simulink model "nnsmc_position_HIL"  (R2024b)
settings: Solver=VariableStepAuto  StartTime=0.0  StopTime=0.005  RelTol=1e-3
undefined symbols (not defined in the file or in its folder): CR, LF
libraries: instrumentseriallib x3, stmutilitieslib x1
settings Model: Creator=mohsen  LastModifiedBy=mohsen

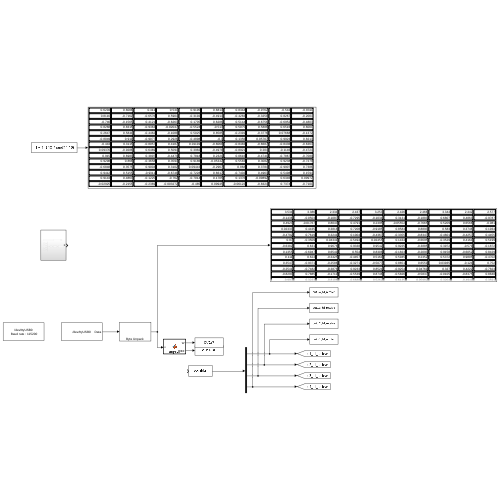
[thumbnail: Simulink's stored preview of the top-level diagram]
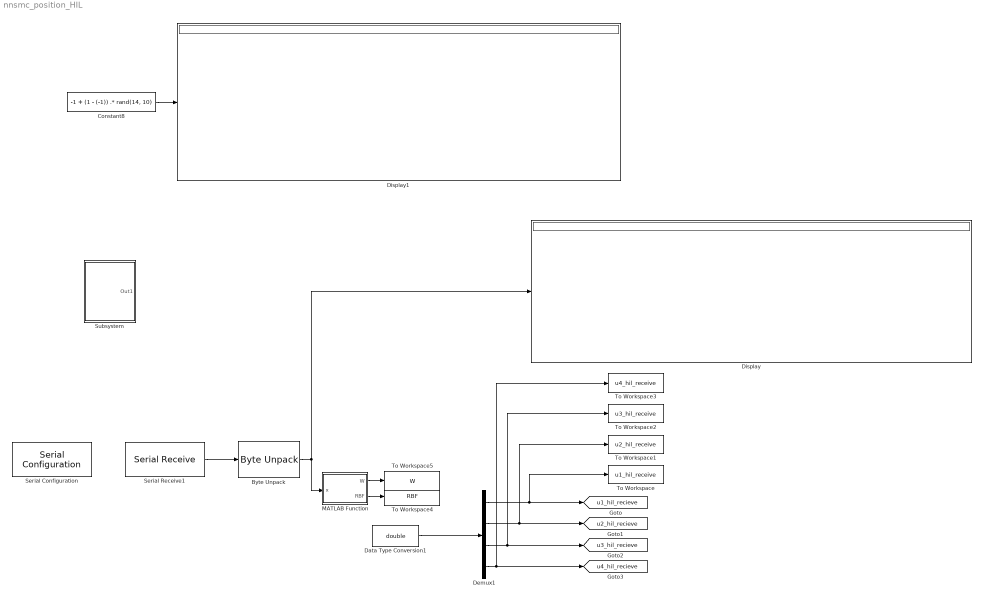
== system nnsmc_position_HIL ==
  Byte Unpack : stmutilitieslib/Byte Unpack  dimensions={[150]}  datatypes={'single'}  byteAlign=1  blockPlatform=stm32f4discovery
  Constant8 : Constant  Value=-1 + (1 - (-1)) .* rand(14, 10)
  Data Type Conversion1 : DataTypeConversion  OutDataTypeStr=double  SaturateOnIntegerOverflow=off  RndMeth=Floor
  Demux1 : Demux
  Display : Display
  Display1 : Display
  MATLAB Function : MATLAB Function  TreatAsAtomicUnit=on
  Serial Configuration : instrumentseriallib/Serial Configuration  Priority=-200000  PortSel=/dev/ttyUSB0  Port=/dev/ttyUSB0  ComPort=/dev/ttyUSB0  BaudRate=115200  DataBits=8  Parity=none  StopBits=1  ByteOrder=little-endian  FlowControl=none  Timeout=0.1  SimulateUsing=Interpreted execution  BlockInModel=on  aMode=1
      settings: LibrarySourceBlock=c2000lib/Host Communication/Serial Configuration
  Serial Receive1 : instrumentseriallib/Serial Receive  Priority=1  PortSel=/dev/ttyUSB0  Port=/dev/ttyUSB0  ComPort=/dev/ttyUSB0  DataType=uint8  SaveDataType=uint8  ToggleHeader=on  Header=[170 187 204]  ToggleDataSize=on  DataSize=600  ToggleTerminator=off  Terminator=CR/LF ('\r\n')  CustomTerminator=[]  InputFormat=Column major  EnableBlockingMode=on  ActionDataUnavailable=Output last received value  ActionWhenDataUnavailable=Output last received value  CustomValue=0  SampleTime=0.005  SimulateUsing=Interpreted execution  BlockInModel=on  aMode=1
      settings: LibrarySourceBlock=c2000lib/Host Communication/Serial Receive
  Subsystem : Subsystem
  To Workspace : ToWorkspace  VariableName=u1_hil_receive  SampleTime=-1
      settings: Save2DSignal=2-D array (concatenate along first dimension)
  To Workspace1 : ToWorkspace  VariableName=u2_hil_receive  SampleTime=-1
      settings: Save2DSignal=2-D array (concatenate along first dimension)
  To Workspace2 : ToWorkspace  VariableName=u3_hil_receive  SampleTime=-1
      settings: Save2DSignal=2-D array (concatenate along first dimension)
  To Workspace3 : ToWorkspace  VariableName=u4_hil_receive  SampleTime=-1
      settings: Save2DSignal=2-D array (concatenate along first dimension)
  To Workspace4 : ToWorkspace  VariableName=RBF  SampleTime=-1
      settings: Save2DSignal=2-D array (concatenate along first dimension)
  To Workspace5 : ToWorkspace  VariableName=W  SampleTime=-1
      settings: Save2DSignal=2-D array (concatenate along first dimension)
  tag scope: u1_hil_recieve=global, u2_hil_recieve=global, u3_hil_recieve=global, u4_hil_recieve=global
  wires:
  Demux1/2 -> To Workspace1/1, [u2_hil_recieve]
  Data Type Conversion1/1 -> Demux1/1
  Demux1/3 -> To Workspace2/1, [u3_hil_recieve]
  Demux1/4 -> To Workspace3/1, [u4_hil_recieve]
  Demux1/1 -> [u1_hil_recieve], To Workspace/1
  Constant8/1 -> Display1/1
  Byte Unpack/1 -> Display/1, MATLAB Function/1(x)
  Serial Receive1/1 -> Byte Unpack/1
  MATLAB Function/2(RBF) -> To Workspace4/1
  MATLAB Function/1(W) -> To Workspace5/1

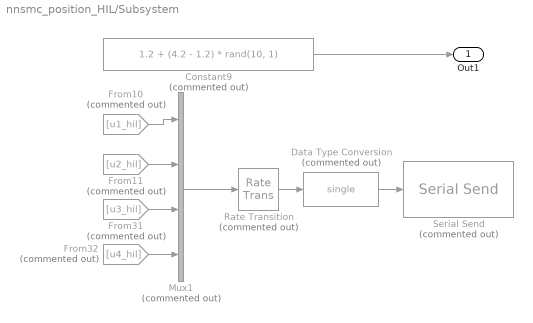
== system nnsmc_position_HIL/Subsystem ==
  Constant9 : Constant  Commented=on  Value=1.2 + (4.2 - 1.2) * rand(10, 1)
  Data Type Conversion : DataTypeConversion  Commented=on  OutDataTypeStr=single  SaturateOnIntegerOverflow=off  RndMeth=Floor
  From10 : From  Commented=on  GotoTag=u1_hil  TagVisibility=global
  From11 : From  Commented=on  GotoTag=u2_hil  TagVisibility=global
  From31 : From  Commented=on  GotoTag=u3_hil  TagVisibility=global
  From32 : From  Commented=on  GotoTag=u4_hil  TagVisibility=global
  Mux1 : Mux  Commented=on
  Rate Transition : RateTransition  Commented=on  OutPortSampleTime=0.005
  Serial Send : instrumentseriallib/Serial Send  Priority=1  Commented=on  PortSel=/dev/ttyUSB0  Port=/dev/ttyUSB0  ComPort=/dev/ttyUSB0  Header=[]  Terminator=<none>  CustomTerminator=[]  EnableBlockingMode=on  SimulateUsing=Interpreted execution  BlockInModel=on  aMode=1
      settings: LibrarySourceBlock=embeddedtargetslib/Host Communication/Serial Send
  Out1 : Outport
  wires:
  Rate Transition/1 -> Data Type Conversion/1
  From31/1 -> Mux1/3
  From10/1 -> Mux1/1
  Constant9/1 -> Out1/1
  From32/1 -> Mux1/4
  From11/1 -> Mux1/2
  Data Type Conversion/1 -> Serial Send/1
  Mux1/1 -> Rate Transition/1

== matlab function nnsmc_position_HIL/MATLAB Function ==
  data: x input; W output; RBF output
function [W, RBF] = unpack(x)

RBF = x(1:10);
W = reshape(x(11:150), [10 14])';
end
